simulink model "INS"  (R2018b)
settings: configuration reference "ins_config" (kept outside this file)
undefined symbols (not defined in the file): DiscIntNeverNeededParam, INS_CONST, INS_EXPORT, INS_PARAM
libraries: simulink x99, AP_Math x15, Filter x6, Quaternion x2, Rotation x2
(part 2 of 4)

== system INS/Sensor_Process/Optical_Flow_Preprocessing/Valid_Detect ==
  timestamp_ms : Inport
  vf_valid : Inport  Port=2
  Compare To Constant4 : simulink/Logic and Bit Operations/Compare To Constant  relop=<  const=100  OutDataTypeStr=uint8
  Constant : Constant  OutDataTypeStr=single
  Detect Change : simulink/Logic and Bit Operations/Detect Change  vinit=0  OutDataTypeStr=boolean
  Discrete-Time Integrator : DiscreteIntegrator  IntegratorMethod=Accumulation: Forward Euler  ExternalReset=sampled level  SampleTime=-1  OutDataTypeStr=uint32  SaturateOnIntegerOverflow=on  ICPrevOutput=DiscIntNeverNeededParam  ICPrevScaledInput=DiscIntNeverNeededParam
  Logical Operator : Logic  AllPortsSameDT=off  OutDataTypeStr=boolean
  valid : Outport
  wires:
  Compare To Constant4/1 -> Logical Operator/1
  Constant/1 -> Discrete-Time Integrator/1
  Detect Change/1 -> Discrete-Time Integrator/2
  vf_valid/1 -> Logical Operator/2
  Discrete-Time Integrator/1 -> Compare To Constant4/1
  Logical Operator/1 -> valid/1
  timestamp_ms/1 -> Detect Change/1

== system INS/Sensor_Process/Sonar_Process/Valid_Check ==
  timestamp_ms : Inport
  diatance_m : Inport  Port=2
  Translation_Data : Inport  Port=3
  Add : Sum
  Bus Selector : BusSelector  OutputSignals=vel_N_mDs,vel_E_mDs
  Compare To Constant : simulink/Logic and Bit Operations/Compare To Constant  relop=<  const=5  OutDataTypeStr=boolean
  Compare To Constant4 : simulink/Logic and Bit Operations/Compare To Constant  relop=<  const=100  OutDataTypeStr=uint8
  Constant : Constant  Value=INS_EXPORT.period  OutDataTypeStr=single
  Constant1 : Constant  OutDataTypeStr=uint8
  Delay : Delay  DelayLength=1
  Detect Change : simulink/Logic and Bit Operations/Detect Change  vinit=0  OutDataTypeStr=boolean
  Discrete-Time Integrator : DiscreteIntegrator  IntegratorMethod=Accumulation: Forward Euler  ExternalReset=sampled level  SampleTime=-1  OutDataTypeStr=uint32  SaturateOnIntegerOverflow=on  ICPrevOutput=DiscIntNeverNeededParam  ICPrevScaledInput=DiscIntNeverNeededParam
  Interval Test : simulink/Logic and Bit Operations/Interval Test  IntervalClosedRight=on  uplimit=2.5  IntervalClosedLeft=off  lowlimit=0  OutDataTypeStr=boolean
  Logical Operator : Logic  Inputs=4  AllPortsSameDT=off  OutDataTypeStr=boolean
  Sqrt : Sqrt  SaturateOnIntegerOverflow=on
  Square : Math  Operator=square  SaturateOnIntegerOverflow=on
  Square1 : Math  Operator=square  SaturateOnIntegerOverflow=on
  Switch : Switch  Criteria=u2 > Threshold
  sonar_valid : Outport
  wires:
  Detect Change/1 -> Switch/2, Discrete-Time Integrator/2
  Discrete-Time Integrator/1 -> Compare To Constant4/1
  Constant/1 -> Discrete-Time Integrator/1
  timestamp_ms/1 -> Detect Change/1
  Logical Operator/1 -> sonar_valid/1
  Constant1/1 -> Switch/1
  Switch/1 -> Delay/1
  Delay/1 -> Logical Operator/2, Switch/3
  Compare To Constant4/1 -> Logical Operator/1  "sonar_valid"
  diatance_m/1 -> Interval Test/1
  Interval Test/1 -> Logical Operator/3
  Translation_Data/1 -> Bus Selector/1
  Bus Selector/1 -> Square/1  "<vel_N_mDs>"
  Bus Selector/2 -> Square1/1  "<vel_E_mDs>"
  Square/1 -> Add/1
  Square1/1 -> Add/2
  Add/1 -> Sqrt/1
  Sqrt/1 -> Compare To Constant/1
  Compare To Constant/1 -> Logical Operator/4

== system INS/Bus_Assignment/Status_Output/INS_Flag/valid_check1 ==
  quality : Inport
  Compare To Constant : simulink/Logic and Bit Operations/Compare To Constant  relop=>=  const=time_out  OutDataTypeStr=boolean
  Compare To Constant1 : simulink/Logic and Bit Operations/Compare To Constant  relop=>  const=0  OutDataTypeStr=boolean
  Compare To Constant2 : simulink/Logic and Bit Operations/Compare To Constant  relop=>  const=0  OutDataTypeStr=boolean
  Constant : Constant  Value=INS_EXPORT.period  OutDataTypeStr=Inherit: Inherit via back propagation
  Delay : Delay  DelayLength=1
  Detect Rise Positive : simulink/Logic and Bit Operations/Detect Rise Positive  vinit=0  OutDataTypeStr=boolean
  Discrete-Time Integrator : DiscreteIntegrator  IntegratorMethod=Accumulation: Forward Euler  gainval=1  ExternalReset=level  SampleTime=-1  ICPrevOutput=DiscIntNeverNeededParam  ICPrevScaledInput=DiscIntNeverNeededParam
  Logical Operator : Logic  Operator=NOT  AllPortsSameDT=off  OutDataTypeStr=boolean
  Logical Operator1 : Logic  Operator=OR  AllPortsSameDT=off  OutDataTypeStr=boolean
  Multiply : Product
  valid : Outport
  wires:
  Multiply/1 -> valid/1
  Delay/1 -> Multiply/2, Logical Operator1/2
  Logical Operator1/1 -> Delay/1
  Detect Rise Positive/1 -> Logical Operator1/1
  Compare To Constant2/1 -> Detect Rise Positive/1
  quality/1 -> Compare To Constant1/1, Compare To Constant2/1
  Compare To Constant1/1 -> Discrete-Time Integrator/2
  Constant/1 -> Discrete-Time Integrator/1
  Discrete-Time Integrator/1 -> Compare To Constant/1
  Compare To Constant/1 -> Logical Operator/1
  Logical Operator/1 -> Multiply/1

== system INS/Bus_Assignment/Status_Output/INS_Flag/valid_check2 ==
  quality : Inport
  Compare To Constant : simulink/Logic and Bit Operations/Compare To Constant  relop=>=  const=time_out  OutDataTypeStr=boolean
  Compare To Constant1 : simulink/Logic and Bit Operations/Compare To Constant  relop=>  const=0  OutDataTypeStr=boolean
  Compare To Constant2 : simulink/Logic and Bit Operations/Compare To Constant  relop=>  const=0  OutDataTypeStr=boolean
  Constant : Constant  Value=INS_EXPORT.period  OutDataTypeStr=Inherit: Inherit via back propagation
  Delay : Delay  DelayLength=1
  Detect Rise Positive : simulink/Logic and Bit Operations/Detect Rise Positive  vinit=0  OutDataTypeStr=boolean
  Discrete-Time Integrator : DiscreteIntegrator  IntegratorMethod=Accumulation: Forward Euler  gainval=1  ExternalReset=level  SampleTime=-1  ICPrevOutput=DiscIntNeverNeededParam  ICPrevScaledInput=DiscIntNeverNeededParam
  Logical Operator : Logic  Operator=NOT  AllPortsSameDT=off  OutDataTypeStr=boolean
  Logical Operator1 : Logic  Operator=OR  AllPortsSameDT=off  OutDataTypeStr=boolean
  Multiply : Product
  valid : Outport
  wires:
  Multiply/1 -> valid/1
  Delay/1 -> Multiply/2, Logical Operator1/2
  Logical Operator1/1 -> Delay/1
  Detect Rise Positive/1 -> Logical Operator1/1
  Compare To Constant2/1 -> Detect Rise Positive/1
  quality/1 -> Compare To Constant1/1, Compare To Constant2/1
  Compare To Constant1/1 -> Discrete-Time Integrator/2
  Constant/1 -> Discrete-Time Integrator/1
  Discrete-Time Integrator/1 -> Compare To Constant/1
  Compare To Constant/1 -> Logical Operator/1
  Logical Operator/1 -> Multiply/1

== system INS/Bus_Assignment/Status_Output/INS_Flag/valid_check3 ==
  quality : Inport
  Compare To Constant : simulink/Logic and Bit Operations/Compare To Constant  relop=>=  const=time_out  OutDataTypeStr=boolean
  Compare To Constant1 : simulink/Logic and Bit Operations/Compare To Constant  relop=>  const=0  OutDataTypeStr=boolean
  Compare To Constant2 : simulink/Logic and Bit Operations/Compare To Constant  relop=>  const=0  OutDataTypeStr=boolean
  Constant : Constant  Value=INS_EXPORT.period  OutDataTypeStr=Inherit: Inherit via back propagation
  Delay : Delay  DelayLength=1
  Detect Rise Positive : simulink/Logic and Bit Operations/Detect Rise Positive  vinit=0  OutDataTypeStr=boolean
  Discrete-Time Integrator : DiscreteIntegrator  IntegratorMethod=Accumulation: Forward Euler  gainval=1  ExternalReset=level  SampleTime=-1  ICPrevOutput=DiscIntNeverNeededParam  ICPrevScaledInput=DiscIntNeverNeededParam
  Logical Operator : Logic  Operator=NOT  AllPortsSameDT=off  OutDataTypeStr=boolean
  Logical Operator1 : Logic  Operator=OR  AllPortsSameDT=off  OutDataTypeStr=boolean
  Multiply : Product
  valid : Outport
  wires:
  Multiply/1 -> valid/1
  Delay/1 -> Multiply/2, Logical Operator1/2
  Logical Operator1/1 -> Delay/1
  Detect Rise Positive/1 -> Logical Operator1/1
  Compare To Constant2/1 -> Detect Rise Positive/1
  quality/1 -> Compare To Constant1/1, Compare To Constant2/1
  Compare To Constant1/1 -> Discrete-Time Integrator/2
  Constant/1 -> Discrete-Time Integrator/1
  Discrete-Time Integrator/1 -> Compare To Constant/1
  Compare To Constant/1 -> Logical Operator/1
  Logical Operator/1 -> Multiply/1

== system INS/Bus_Assignment/Status_Output/INS_Flag/valid_check4 ==
  quality : Inport
  Compare To Constant : simulink/Logic and Bit Operations/Compare To Constant  relop=>=  const=time_out  OutDataTypeStr=boolean
  Compare To Constant1 : simulink/Logic and Bit Operations/Compare To Constant  relop=>  const=0  OutDataTypeStr=boolean
  Compare To Constant2 : simulink/Logic and Bit Operations/Compare To Constant  relop=>  const=0  OutDataTypeStr=boolean
  Constant : Constant  Value=INS_EXPORT.period  OutDataTypeStr=Inherit: Inherit via back propagation
  Delay : Delay  DelayLength=1
  Detect Rise Positive : simulink/Logic and Bit Operations/Detect Rise Positive  vinit=0  OutDataTypeStr=boolean
  Discrete-Time Integrator : DiscreteIntegrator  IntegratorMethod=Accumulation: Forward Euler  gainval=1  ExternalReset=level  SampleTime=-1  ICPrevOutput=DiscIntNeverNeededParam  ICPrevScaledInput=DiscIntNeverNeededParam
  Logical Operator : Logic  Operator=NOT  AllPortsSameDT=off  OutDataTypeStr=boolean
  Logical Operator1 : Logic  Operator=OR  AllPortsSameDT=off  OutDataTypeStr=boolean
  Multiply : Product
  valid : Outport
  wires:
  Multiply/1 -> valid/1
  Delay/1 -> Multiply/2, Logical Operator1/2
  Logical Operator1/1 -> Delay/1
  Detect Rise Positive/1 -> Logical Operator1/1
  Compare To Constant2/1 -> Detect Rise Positive/1
  quality/1 -> Compare To Constant1/1, Compare To Constant2/1
  Compare To Constant1/1 -> Discrete-Time Integrator/2
  Constant/1 -> Discrete-Time Integrator/1
  Discrete-Time Integrator/1 -> Compare To Constant/1
  Compare To Constant/1 -> Logical Operator/1
  Logical Operator/1 -> Multiply/1

== system INS/Bus_Assignment/Status_Output/INS_Flag/valid_check5 ==
  quality : Inport
  Compare To Constant : simulink/Logic and Bit Operations/Compare To Constant  relop=>=  const=time_out  OutDataTypeStr=boolean
  Compare To Constant1 : simulink/Logic and Bit Operations/Compare To Constant  relop=>  const=0  OutDataTypeStr=boolean
  Compare To Constant2 : simulink/Logic and Bit Operations/Compare To Constant  relop=>  const=0  OutDataTypeStr=boolean
  Constant : Constant  Value=INS_EXPORT.period  OutDataTypeStr=Inherit: Inherit via back propagation
  Delay : Delay  DelayLength=1
  Detect Rise Positive : simulink/Logic and Bit Operations/Detect Rise Positive  vinit=0  OutDataTypeStr=boolean
  Discrete-Time Integrator : DiscreteIntegrator  IntegratorMethod=Accumulation: Forward Euler  gainval=1  ExternalReset=level  SampleTime=-1  ICPrevOutput=DiscIntNeverNeededParam  ICPrevScaledInput=DiscIntNeverNeededParam
  Logical Operator : Logic  Operator=NOT  AllPortsSameDT=off  OutDataTypeStr=boolean
  Logical Operator1 : Logic  Operator=OR  AllPortsSameDT=off  OutDataTypeStr=boolean
  Multiply : Product
  valid : Outport
  wires:
  Multiply/1 -> valid/1
  Delay/1 -> Multiply/2, Logical Operator1/2
  Logical Operator1/1 -> Delay/1
  Detect Rise Positive/1 -> Logical Operator1/1
  Compare To Constant2/1 -> Detect Rise Positive/1
  quality/1 -> Compare To Constant1/1, Compare To Constant2/1
  Compare To Constant1/1 -> Discrete-Time Integrator/2
  Constant/1 -> Discrete-Time Integrator/1
  Discrete-Time Integrator/1 -> Compare To Constant/1
  Compare To Constant/1 -> Logical Operator/1
  Logical Operator/1 -> Multiply/1

== system INS/Bus_Assignment/Status_Output/INS_Flag/valid_check6 ==
  quality : Inport
  Compare To Constant : simulink/Logic and Bit Operations/Compare To Constant  relop=>=  const=time_out  OutDataTypeStr=boolean
  Compare To Constant1 : simulink/Logic and Bit Operations/Compare To Constant  relop=>  const=0  OutDataTypeStr=boolean
  Compare To Constant2 : simulink/Logic and Bit Operations/Compare To Constant  relop=>  const=0  OutDataTypeStr=boolean
  Constant : Constant  Value=INS_EXPORT.period  OutDataTypeStr=Inherit: Inherit via back propagation
  Delay : Delay  DelayLength=1
  Detect Rise Positive : simulink/Logic and Bit Operations/Detect Rise Positive  vinit=0  OutDataTypeStr=boolean
  Discrete-Time Integrator : DiscreteIntegrator  IntegratorMethod=Accumulation: Forward Euler  gainval=1  ExternalReset=level  SampleTime=-1  ICPrevOutput=DiscIntNeverNeededParam  ICPrevScaledInput=DiscIntNeverNeededParam
  Logical Operator : Logic  Operator=NOT  AllPortsSameDT=off  OutDataTypeStr=boolean
  Logical Operator1 : Logic  Operator=OR  AllPortsSameDT=off  OutDataTypeStr=boolean
  Multiply : Product
  valid : Outport
  wires:
  Multiply/1 -> valid/1
  Delay/1 -> Multiply/2, Logical Operator1/2
  Logical Operator1/1 -> Delay/1
  Detect Rise Positive/1 -> Logical Operator1/1
  Compare To Constant2/1 -> Detect Rise Positive/1
  quality/1 -> Compare To Constant1/1, Compare To Constant2/1
  Compare To Constant1/1 -> Discrete-Time Integrator/2
  Constant/1 -> Discrete-Time Integrator/1
  Discrete-Time Integrator/1 -> Compare To Constant/1
  Compare To Constant/1 -> Logical Operator/1
  Logical Operator/1 -> Multiply/1

== system INS/Bus_Assignment/Status_Output/INS_Flag/valid_check8 ==
  quality : Inport
  Compare To Constant : simulink/Logic and Bit Operations/Compare To Constant  relop=>=  const=time_out  OutDataTypeStr=boolean
  Compare To Constant1 : simulink/Logic and Bit Operations/Compare To Constant  relop=>  const=0  OutDataTypeStr=boolean
  Compare To Constant2 : simulink/Logic and Bit Operations/Compare To Constant  relop=>  const=0  OutDataTypeStr=boolean
  Constant : Constant  Value=INS_EXPORT.period  OutDataTypeStr=Inherit: Inherit via back propagation
  Delay : Delay  DelayLength=1
  Detect Rise Positive : simulink/Logic and Bit Operations/Detect Rise Positive  vinit=0  OutDataTypeStr=boolean
  Discrete-Time Integrator : DiscreteIntegrator  IntegratorMethod=Accumulation: Forward Euler  gainval=1  ExternalReset=level  SampleTime=-1  ICPrevOutput=DiscIntNeverNeededParam  ICPrevScaledInput=DiscIntNeverNeededParam
  Logical Operator : Logic  Operator=NOT  AllPortsSameDT=off  OutDataTypeStr=boolean
  Logical Operator1 : Logic  Operator=OR  AllPortsSameDT=off  OutDataTypeStr=boolean
  Multiply : Product
  valid : Outport
  wires:
  Multiply/1 -> valid/1
  Delay/1 -> Multiply/2, Logical Operator1/2
  Logical Operator1/1 -> Delay/1
  Detect Rise Positive/1 -> Logical Operator1/1
  Compare To Constant2/1 -> Detect Rise Positive/1
  quality/1 -> Compare To Constant1/1, Compare To Constant2/1
  Compare To Constant1/1 -> Discrete-Time Integrator/2
  Constant/1 -> Discrete-Time Integrator/1
  Discrete-Time Integrator/1 -> Compare To Constant/1
  Compare To Constant/1 -> Logical Operator/1
  Logical Operator/1 -> Multiply/1

== system INS/Data_Fusion/AHRS/Attitude_Init/Attitude_Init ==
  acc_B : Inport
  mag_B : Inport  Port=2
  Enable : EnablePort
  DCM_to_quat : Quaternion/DCM_to_quat  SystemSampleTime=-1
  Gain : Gain  Gain=-1
  Vector Concatenate : Concatenate  NumInputs=3  Mode=Multidimensional array  ConcatenateDimension=2
  cross_product : AP_Math/cross_product  SystemSampleTime=-1
  cross_product1 : AP_Math/cross_product  SystemSampleTime=-1
  safe_norm : AP_Math/safe_norm  SystemSampleTime=-1
  safe_norm1 : AP_Math/safe_norm  SystemSampleTime=-1
  safe_norm2 : AP_Math/safe_norm  SystemSampleTime=-1
  quaternion_0 : Outport  InitialOutput=[1; 0; 0; 0]
  wires:
  Gain/1 -> cross_product/1, safe_norm2/1, cross_product1/2
  acc_B/1 -> Gain/1
  Vector Concatenate/1 -> DCM_to_quat/1  "M_BO"
  cross_product1/1 -> safe_norm/1
  mag_B/1 -> cross_product/2
  cross_product/1 -> cross_product1/1, safe_norm1/1
  safe_norm1/1 -> Vector Concatenate/2  "DCM_y"
  safe_norm/1 -> Vector Concatenate/1  "DCM_x"
  safe_norm2/1 -> Vector Concatenate/3  "DCM_z"
  DCM_to_quat/1 -> quaternion_0/1

== system INS/Data_Fusion/AHRS/Attitude_Init/Onground_Check ==
  IMU_Data : Inport
  Abs : Abs
  Bus Selector : BusSelector  OutputSignals=gyr_B_radPs
  HPF : Subsystem
  LPF : Filter/LPF  T=0.5
  LPF1 : Filter/LPF  T=0.05
  MinMax1 : MinMax  Function=max
  Relay2 : Relay  OnSwitchValue=10e-3  OffSwitchValue=3e-3  OnOutputValue=0  OffOutputValue=1
  Saturation2 : Saturate  UpperLimit=1  LowerLimit=0
  Selector : Selector  InputPortWidth=3  IndexOptions=Index vector (dialog)  Indices=[1 2]  OutputSizes=1
  standstill : Outport
  wires:
  LPF1/1 -> Relay2/1
  Relay2/1 -> standstill/1
  Saturation2/1 -> LPF1/1
  HPF/1(y) -> Abs/1
  Selector/1 -> HPF/1(u)
  Abs/1 -> MinMax1/1
  LPF/1 -> Saturation2/1
  MinMax1/1 -> LPF/1  "gyr_sig"
  Bus Selector/1 -> Selector/1  "<gyr_B_radPs>"
  IMU_Data/1 -> Bus Selector/1

== system INS/Data_Fusion/AHRS/Attitude_Init/Reset_Condition ==
  IMU_valid : Inport
  Mag_valid : Inport  Port=2
  global_reset : Inport  Port=3
  acc_B_mPs2 : Inport  Port=4
  mag_norm_B : Inport  Port=5
  Compare To Constant : simulink/Logic and Bit Operations/Compare To Constant  relop=>  const=0.01  OutDataTypeStr=boolean
  Interval Test : simulink/Logic and Bit Operations/Interval Test  IntervalClosedRight=on  uplimit=INS_CONST.g+0.5  IntervalClosedLeft=on  lowlimit=INS_CONST.g-0.5  OutDataTypeStr=boolean
  Logical Operator : Logic  Operator=OR  AllPortsSameDT=off  OutDataTypeStr=boolean
  Logical Operator1 : Logic  Inputs=4  AllPortsSameDT=off  OutDataTypeStr=boolean
  reset : Subsystem
  vec_modulus : AP_Math/vec_modulus  SystemSampleTime=-1
  vec_modulus1 : AP_Math/vec_modulus  SystemSampleTime=-1
  att_reset : Outport
  wires:
  IMU_valid/1 -> Logical Operator1/1
  reset/1(reset) -> Logical Operator/1  "a_reset"
  global_reset/1 -> Logical Operator/2
  Logical Operator/1 -> att_reset/1
  Mag_valid/1 -> Logical Operator1/2
  acc_B_mPs2/1 -> vec_modulus/1
  mag_norm_B/1 -> vec_modulus1/1
  vec_modulus1/1 -> Compare To Constant/1
  Compare To Constant/1 -> Logical Operator1/4
  Interval Test/1 -> Logical Operator1/3
  vec_modulus/1 -> Interval Test/1
  Logical Operator1/1 -> reset/1(valid)  "a_valid"

== system INS/Data_Fusion/AHRS/Correct/Att_Correction ==
  Sensor_Data : Inport
  Rotation_Data : Inport  Port=2
  standstill : Inport  Port=3
  Attitude_Correct : Subsystem
  Bus Selector : BusSelector  OutputSignals=Mag_Data,GPS_Data
  Bus Selector2 : BusSelector  OutputSignals=M_BO
  Heading_Correction : Subsystem
  Multiply : Product  Multiplication=Matrix(*)
  Sum : Sum  Inputs=|++
  rot_B_correction : Outport
  wires:
  standstill/1 -> Heading_Correction/2(standstill)
  Bus Selector/1 -> Heading_Correction/3(Mag_Data)  "<Mag_Data>"
  Attitude_Correct/1(att_error_O_mPs2) -> Sum/1  "att_error_O"
  Heading_Correction/1(heading_error_O) -> Sum/2  "heading_error_O"
  Bus Selector2/1 -> Multiply/1  "<M_BO>"
  Multiply/1 -> rot_B_correction/1
  Sensor_Data/1 -> Bus Selector/1, Attitude_Correct/1(Sensor_Data)
  Sum/1 -> Multiply/2
  Bus Selector/2 -> Heading_Correction/4(GPS_Data)  "<GPS_Data>"
  Rotation_Data/1 -> Bus Selector2/1, Heading_Correction/1(Rotation_Data), Attitude_Correct/2(Rotation_Data)

== system INS/Data_Fusion/AHRS/Correct/Bias_Correction ==
  rot_B_correction : Inport
  Rotation_Data : Inport  Port=2
  standstill : Inport  Port=3
  IMU_Data : Inport  Port=4
  Abs : Abs
  Bus Selector : BusSelector  OutputSignals=acc_B_mPs2
  Bus Selector1 : BusSelector  OutputSignals=gyr_B_radDs
  Compare To Constant : simulink/Logic and Bit Operations/Compare To Constant  relop=<=  const=1  OutDataTypeStr=boolean
  Constant : Constant  Value=9.806  OutDataTypeStr=single
  Data Type Conversion : DataTypeConversion  OutDataTypeStr=single
  Gain3 : Gain  Gain=0.5
  Gain4 : Gain
  MX Product1 : Product  RndMeth=Simplest
  Onground_Correction : Subsystem
  Saturation2 : Saturate  UpperLimit=0.1/180*pi  LowerLimit=-0.1/180*pi
  Subtract : Sum  Inputs=+-
  Sum2 : Sum  Inputs=|+-
  vec_modulus : AP_Math/vec_modulus  SystemSampleTime=-1
  bias_g_correction : Outport
  wires:
  Bus Selector1/1 -> Onground_Correction/1(gyr_B_radPs)  "<gyr_B_radDs>"
  Rotation_Data/1 -> Bus Selector1/1
  standstill/1 -> Onground_Correction/2(standstill)
  IMU_Data/1 -> Bus Selector/1
  Saturation2/1 -> Sum2/1  "bias_g_correction"
  Compare To Constant/1 -> Data Type Conversion/1
  Bus Selector/1 -> vec_modulus/1  "<acc_B_mPs2>"
  MX Product1/1 -> Gain3/1
  rot_B_correction/1 -> MX Product1/1
  vec_modulus/1 -> Subtract/1
  Gain3/1 -> Saturation2/1
  Onground_Correction/1(gyr_bias) -> Gain4/1
  Gain4/1 -> Sum2/2  "rot_bias_standstil"
  Constant/1 -> Subtract/2
  Subtract/1 -> Abs/1
  Abs/1 -> Compare To Constant/1
  Data Type Conversion/1 -> MX Product1/2
  Sum2/1 -> bias_g_correction/1  "bias_g_correction"

== system INS/Data_Fusion/AHRS/Integrate/Att_Init_Done ==
  att_reset : Inport
  Constant : Constant  OutDataTypeStr=uint8
  Delay : Delay  DelayLength=1
  Detect Increase : simulink/Logic and Bit Operations/Detect Increase  vinit=0.0  OutDataTypeStr=boolean
  Switch : Switch  Criteria=u2 > Threshold
  att_init_done : Outport
  wires:
  att_reset/1 -> Detect Increase/1
  Detect Increase/1 -> Switch/2
  Constant/1 -> Switch/1
  Delay/1 -> Switch/3
  Switch/1 -> att_init_done/1, Delay/1

== system INS/Data_Fusion/AHRS/Integrate/Attitude_Integration ==
  att_reset : Inport
  quat_0 : Inport  Port=2
  rot_IB_B : Inport  Port=3
  Constant : Constant  Value=0  OutDataTypeStr=single
  Discrete-Time Integrator : DiscreteIntegrator  ExternalReset=level  InitialConditionSource=external  SampleTime=-1  ICPrevOutput=DiscIntNeverNeededParam  ICPrevScaledInput=DiscIntNeverNeededParam
  Gain2 : Gain  Gain=0.5  OutMin=-450*pi/180  OutMax=450*pi/180  RndMeth=Simplest
  Mux1 : Mux  Inputs=2
  Quat Multiply1 : Subsystem  mask(Quaternion Multiplication){}
      mask help:
      | q(1) = q1(1)*q2(1) - q1(2)*q2(2) - q1(3)*q2(3) - q1(4)*q2(4)
      | q(2) = q1(1)*q2(2) + q1(2)*q2(1) + q1(3)*q2(4) - q1(4)*q2(3)
      | q(3) = q1(1)*q2(3) - q1(2)*q2(4) + q1(3)*q2(1) + q1(4)*q2(2)
      | q(4) = q1(1)*q2(4) + q1(2)*q2(3) - q1(3)*q2(2) + q1(4)*q2(1)
      |
      | Regrettably implemented in Simulink
      mask init:
      | pos = get_param(gcb, 'Position');
      | width = pos(3) - pos(1); height = pos(4) - pos(2);
      | fontsize = get_param(gcb, 'fontsize');
      | if fontsize==-1, scale=1; else scale=fontsize/10; end
      mask Display: text(width/2-scale*14, (height/2-scale), 'q1*q2')
  Quat_to_M_OB : Rotation/Quat_to_M_OB  SystemSampleTime=-1
  Transpose2 : Math  Operator=transpose  SaturateOnIntegerOverflow=on
  quat normalize : Quaternion/quat normalize  SystemSampleTime=-1
  att_quat : Outport
  M_OB : Outport  Port=2
  M_BO : Outport  Port=3
  wires:
  Transpose2/1 -> M_BO/1
  Quat_to_M_OB/1 -> M_OB/1, Transpose2/1
  Discrete-Time Integrator/1 -> quat normalize/1
  att_reset/1 -> Discrete-Time Integrator/2
  quat_0/1 -> Discrete-Time Integrator/3
  Gain2/1 -> Discrete-Time Integrator/1
  Quat Multiply1/1(q) -> Gain2/1
  rot_IB_B/1 -> Mux1/2
  Mux1/1 -> Quat Multiply1/2(q2)
  Constant/1 -> Mux1/1
  quat normalize/1 -> Quat_to_M_OB/1, Quat Multiply1/1(q1), att_quat/1

== system INS/Data_Fusion/AHRS/Integrate/Bias_Integration ==
  bias_g_correction : Inport
  rot_IB_B : Inport  Port=2
  Discrete-Time Integrator2 : DiscreteIntegrator  SampleTime=-1  LimitOutput=on  UpperSaturationLimit=50/180*pi  LowerSaturationLimit=-50/180*pi  ICPrevOutput=DiscIntNeverNeededParam  ICPrevScaledInput=DiscIntNeverNeededParam
  Sum1 : Sum  Inputs=++|
  rot_B_cal_radDs : Outport
  bias_g : Outport  Port=2
  wires:
  bias_g_correction/1 -> Discrete-Time Integrator2/1
  Sum1/1 -> rot_B_cal_radDs/1
  Discrete-Time Integrator2/1 -> Sum1/1, bias_g/1
  rot_IB_B/1 -> Sum1/2

== system INS/Data_Fusion/AHRS/Integrate/Euler_Angle ==
  att_quat : Inport
  M_BO : Inport  Port=2
  Euler_Transformations : Subsystem
  M_CO1 : Rotation/M_CO  SystemSampleTime=-1
  Selector2 : Selector  NumberOfDimensions=2  InputPortWidth=3  IndexOptions=Index vector (dialog),Index vector (dialog)  Indices=[1 2 3],[3]  OutputSizes=1,1
  phi_rad : Outport
  theta_rad : Outport  Port=2
  psi_rad : Outport  Port=3
  M_CO : Outport  Port=4
  wires:
  Euler_Transformations/1(phi_rad) -> phi_rad/1
  Euler_Transformations/2(theta_rad) -> theta_rad/1
  Euler_Transformations/3(psi_rad) -> M_CO1/1, psi_rad/1
  M_CO1/1 -> M_CO/1
  M_BO/1 -> Selector2/1
  Selector2/1 -> Euler_Transformations/1(Oz_B)
  att_quat/1 -> Euler_Transformations/2(quat_OB)

== system INS/Data_Fusion/Translation_Filter/CF/Bus_Assignment ==
  Processed_Data : Inport
  Horizontal_States : Inport  Port=2
  Verticle_States : Inport  Port=3
  sonar_bias : Inport  Port=4
  Bus Creator : BusCreator  Inputs=12
  Constant : Constant  OutDataTypeStr=Inherit: Inherit via back propagation
  Demux1 : Demux  Outputs=3
  Demux2 : Demux  Outputs=3
  Signal_Rounting : Subsystem
  Translation_Data : Outport
  wires:
  Bus Creator/1 -> Translation_Data/1
  Demux1/3 -> Bus Creator/6  "vel_D_mDs"
  Demux1/2 -> Bus Creator/5  "vel_E_mDs"
  Demux1/1 -> Bus Creator/4  "vel_N_mDs"
  Demux2/3 -> Bus Creator/3  "h_m"
  Demux2/2 -> Bus Creator/2  "lambda_rad"
  Demux2/1 -> Bus Creator/1  "mue_rad"
  Signal_Rounting/3(ba_O_mDs2) -> Bus Creator/7  "ba_O_mDs2"
  Signal_Rounting/2(vel_O_mDs) -> Demux1/1
  Signal_Rounting/1(WGS84_Pos) -> Demux2/1
  Verticle_States/1 -> Signal_Rounting/3(Verticle_States)
  Horizontal_States/1 -> Signal_Rounting/2(Horizontal_States)
  Processed_Data/1 -> Signal_Rounting/1(Processed_Data)
  Constant/1 -> Bus Creator/12  "init_done"
  Signal_Rounting/4(h_gnd_m) -> Bus Creator/8  "h_gnd_m"
  sonar_bias/1 -> Signal_Rounting/4(sonar_bias)
  Signal_Rounting/7(h_R_m) -> Bus Creator/11  "h_R_m"
  Signal_Rounting/5(x_R_m) -> Bus Creator/9  "x_R_m"
  Signal_Rounting/6(y_R_m) -> Bus Creator/10  "y_R_m"

== system INS/Data_Fusion/Translation_Filter/CF/Horizontal_Filter ==
  Processed_Data : Inport
  Rotation_Data : Inport  Port=2
  Correct : Subsystem
  Predict : Subsystem
  Reshape : Reshape  OutputDimensionality=Customize  OutputDimensions=[6,1]
  States : Outport
  wires:
  Predict/1(X_Predict) -> Correct/1(X_Predict)
  Correct/1(X_Next) -> Reshape/1
  Reshape/1 -> Predict/1(X_Prio), States/1
  Processed_Data/1 -> Correct/2(Processed_Data), Predict/3(Processed_Data)
  Rotation_Data/1 -> Predict/2(Rotation_Data)

== system INS/Data_Fusion/Translation_Filter/CF/Verticle_Filter ==
  Processed_Data : Inport
  Rotation_Data : Inport  Port=2
  Correct : Subsystem
  Predict : Subsystem
  Reshape : Reshape  OutputDimensionality=Customize  OutputDimensions=[3,1]
  States : Outport
  wires:
  Predict/1(X_Predict) -> Correct/1(X_Predict)
  Correct/1(X_Next) -> Reshape/1
  Reshape/1 -> Predict/1(X_Prio), States/1
  Processed_Data/1 -> Correct/2(Processed_Data), Predict/3(Processed_Data)
  Rotation_Data/1 -> Predict/2(Rotation_Data)

== system INS/Data_Fusion/Translation_Filter/Process/Process_Data ==
  Sensor_Status : Inport
  Sensor_Meas : Inport  Port=2
  Rotation_Data : Inport  Port=3
  Translation_Data : Inport  Port=4
  Bus Creator : BusCreator  Inputs=4
  Bus Selector : BusSelector  OutputSignals=global_reset
  Init_Condition : Subsystem
  Sensor_Enable : Subsystem
  Sensor_Valid : Subsystem
  Proecssed_Data : Outport
  wires:
  Sensor_Enable/1(Sensor_Enable) -> Bus Creator/1  "Sensor_Enable"
  Init_Condition/1(Init_Condition) -> Bus Creator/2  "Init_Condition"
  Bus Creator/1 -> Proecssed_Data/1
  Rotation_Data/1 -> Init_Condition/4(Rotation_Data)
  Sensor_Meas/1 -> Bus Creator/3, Init_Condition/3(Sensor_Meas)  "Sensor_Meas"
  Sensor_Valid/1(Validity) -> Init_Condition/1(Validity)
  Sensor_Status/1 -> Sensor_Enable/1(Sensor_Status), Sensor_Valid/1(Sensor_Status), Bus Creator/4, Bus Selector/1  "Sensor_Status"
  Bus Selector/1 -> Init_Condition/2(global_reset)  "<global_reset>"
  Translation_Data/1 -> Init_Condition/5(Translation_Data)

== system INS/Data_Fusion/Translation_Filter/Process/Sensor_Meas ==
  Sensor_Data : Inport
  Rotation_Data : Inport  Port=2
  Baro_Process : Subsystem
  Bus Creator : BusCreator  Inputs=4
  GPS_Process : Subsystem
  OpticalFlow_Process : Subsystem
  Sonar_Process : Subsystem
  Sensor_Meas : Outport
  wires:
  Bus Creator/1 -> Sensor_Meas/1
  Sensor_Data/1 -> GPS_Process/1(Sensor_Data), Sonar_Process/1(Sensor_Data), OpticalFlow_Process/1(Sensor_Data), Baro_Process/1(Sensor_Data)
  GPS_Process/1(GPS_Meas) -> Bus Creator/1  "GPS_Meas"
  Rotation_Data/1 -> Sonar_Process/2(Rotation_Data)
  Sonar_Process/1(Sonar_Meas) -> Bus Creator/2  "Sonar_Meas"
  Baro_Process/1(Baro_Meas) -> Bus Creator/3  "Baro_Meas"
  OpticalFlow_Process/1(OptFlow_Meas) -> Bus Creator/4  "OptFlow_Meas"

== system INS/Data_Fusion/Translation_Filter/Process/Sensor_Status ==
  Sensor_Data : Inport
  Baro_Status : Subsystem
  Bus Creator : BusCreator  Inputs=5
  Bus Selector : BusSelector  OutputSignals=global_reset
  GPS_Status : Subsystem
  OpticalFlow_Status : Subsystem
  Sonar_Status : Subsystem
  Sensor_Status : Outport
  wires:
  Bus Creator/1 -> Sensor_Status/1
  Sensor_Data/1 -> GPS_Status/1(Sensor_Data), OpticalFlow_Status/1(Sensor_Data), Bus Selector/1, Baro_Status/1(Sensor_Data), Sonar_Status/1(Sensor_Data)
  GPS_Status/1(GPS_Status) -> Bus Creator/1  "GPS_Status"
  Bus Selector/1 -> Bus Creator/5  "<global_reset>"
  Sonar_Status/1(Sonar_Status) -> Bus Creator/2  "Sonar_Status"
  Baro_Status/1(Baro_Status) -> Bus Creator/3  "Baro_Status"
  OpticalFlow_Status/1(OptFlow_Status) -> Bus Creator/4  "OptFlow_Status"

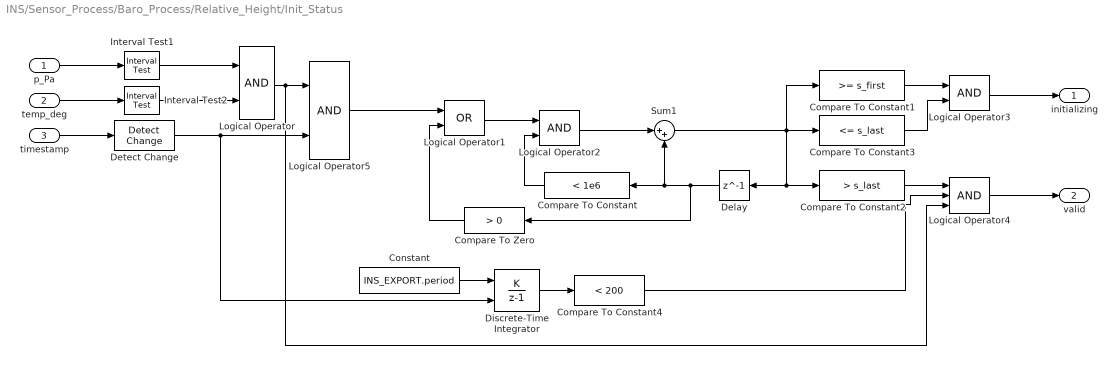
== system INS/Sensor_Process/Baro_Process/Relative_Height/Init_Status ==
  p_Pa : Inport
  temp_deg : Inport  Port=2
  timestamp : Inport  Port=3
  Compare To Constant : simulink/Logic and Bit Operations/Compare To Constant  relop=<  const=1e6  OutDataTypeStr=boolean
  Compare To Constant1 : simulink/Logic and Bit Operations/Compare To Constant  relop=>=  const=s_first  OutDataTypeStr=boolean
  Compare To Constant2 : simulink/Logic and Bit Operations/Compare To Constant  relop=>  const=s_last  OutDataTypeStr=boolean
  Compare To Constant3 : simulink/Logic and Bit Operations/Compare To Constant  relop=<=  const=s_last  OutDataTypeStr=boolean
  Compare To Constant4 : simulink/Logic and Bit Operations/Compare To Constant  relop=<  const=200  OutDataTypeStr=boolean
  Compare To Zero : simulink/Logic and Bit Operations/Compare To Zero  relop=>  OutDataTypeStr=boolean
  Constant : Constant  Value=INS_EXPORT.period  OutDataTypeStr=single
  Delay : Delay  DelayLength=1
  Detect Change : simulink/Logic and Bit Operations/Detect Change  vinit=0  OutDataTypeStr=boolean
  Discrete-Time Integrator : DiscreteIntegrator  IntegratorMethod=Accumulation: Forward Euler  ExternalReset=sampled level  SampleTime=-1  OutDataTypeStr=uint32  SaturateOnIntegerOverflow=on  ICPrevOutput=DiscIntNeverNeededParam  ICPrevScaledInput=DiscIntNeverNeededParam
  Interval Test1 : simulink/Logic and Bit Operations/Interval Test  IntervalClosedRight=off  uplimit=pressure_max  IntervalClosedLeft=off  lowlimit=pressure_min  OutDataTypeStr=boolean
  Interval Test2 : simulink/Logic and Bit Operations/Interval Test  IntervalClosedRight=off  uplimit=temp_max  IntervalClosedLeft=off  lowlimit=temp_min  OutDataTypeStr=boolean
  Logical Operator{,2..3,5} (4 alike) : Logic  AllPortsSameDT=off  OutDataTypeStr=boolean
  Logical Operator1 : Logic  Operator=OR  AllPortsSameDT=off  OutDataTypeStr=boolean
  Logical Operator4 : Logic  Inputs=3  AllPortsSameDT=off  OutDataTypeStr=boolean
  Sum1 : Sum  Inputs=|++  AccumDataTypeStr=uint32  OutDataTypeStr=uint32  RndMeth=Simplest  SaturateOnIntegerOverflow=on
  initializing : Outport
  valid : Outport  Port=2
  wires:
  Logical Operator/1 -> Logical Operator4/3, Logical Operator5/1
  Logical Operator4/1 -> valid/1
  Compare To Constant4/1 -> Logical Operator4/2
  Discrete-Time Integrator/1 -> Compare To Constant4/1
  Detect Change/1 -> Discrete-Time Integrator/2, Logical Operator5/2
  Constant/1 -> Discrete-Time Integrator/1
  Logical Operator3/1 -> initializing/1
  Compare To Constant3/1 -> Logical Operator3/2
  Compare To Constant1/1 -> Logical Operator3/1
  Compare To Constant2/1 -> Logical Operator4/1
  Compare To Constant/1 -> Logical Operator2/2
  Logical Operator1/1 -> Logical Operator2/1
  Compare To Zero/1 -> Logical Operator1/2
  Logical Operator2/1 -> Sum1/1
  Logical Operator5/1 -> Logical Operator1/1
  Sum1/1 -> Compare To Constant3/1, Compare To Constant1/1, Delay/1, Compare To Constant2/1
  Delay/1 -> Compare To Zero/1, Sum1/2, Compare To Constant/1
  Interval Test2/1 -> Logical Operator/2
  temp_deg/1 -> Interval Test2/1
  timestamp/1 -> Detect Change/1
  p_Pa/1 -> Interval Test1/1
  Interval Test1/1 -> Logical Operator/1

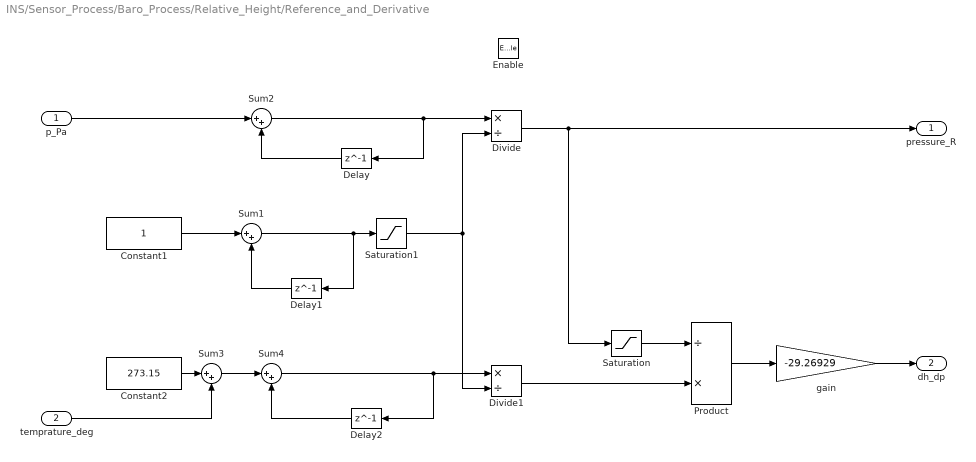
== system INS/Sensor_Process/Baro_Process/Relative_Height/Reference_and_Derivative ==
  p_Pa : Inport
  temprature_deg : Inport  Port=2
  Enable : EnablePort  StatesWhenEnabling=reset
  Constant1 : Constant  OutDataTypeStr=uint32
  Constant2 : Constant  Value=273.15  OutDataTypeStr=single
  Delay : Delay  DelayLength=1
  Delay1 : Delay  DelayLength=1
  Delay2 : Delay  DelayLength=1
  Divide : Product  Inputs=*/
  Divide1 : Product  Inputs=*/
  Product : Product  Inputs=/*
  Saturation : Saturate  UpperLimit=1200e2  LowerLimit=500
  Saturation1 : Saturate  UpperLimit=2^32  LowerLimit=1
  Sum1 : Sum  Inputs=|++  AccumDataTypeStr=uint32  OutDataTypeStr=uint32  RndMeth=Simplest  SaturateOnIntegerOverflow=on
  Sum2 : Sum  Inputs=|++
  Sum3 : Sum  Inputs=|++
  Sum4 : Sum  Inputs=|++
  gain : Gain  Gain=-29.26929
  pressure_R : Outport
  dh_dp : Outport  Port=2
  wires:
  Saturation1/1 -> Divide1/2, Divide/2
  Constant1/1 -> Sum1/1
  Sum1/1 -> Delay1/1, Saturation1/1
  Delay1/1 -> Sum1/2
  Saturation/1 -> Product/1
  Sum2/1 -> Delay/1, Divide/1
  Delay/1 -> Sum2/2
  p_Pa/1 -> Sum2/1
  Divide/1 -> pressure_R/1, Saturation/1
  Constant2/1 -> Sum3/1
  temprature_deg/1 -> Sum3/2
  Sum3/1 -> Sum4/1
  Product/1 -> gain/1
  gain/1 -> dh_dp/1
  Sum4/1 -> Delay2/1, Divide1/1
  Delay2/1 -> Sum4/2
  Divide1/1 -> Product/2

== system INS/Sensor_Process/GPS_Process/GPS_Status_and_Quality/GPS_Status ==
  note: GPS Status
      | 0: idle
      | 1: initialized, but 3D fix lost
      | 2: initialized, with 3D fix
  timeout : Inport
  hAcc : Inport  Port=2
  fixtype : Inport  Port=3
  Compare To Constant : simulink/Logic and Bit Operations/Compare To Constant  relop=<  const=5*1e3  OutDataTypeStr=uint8
  Compare To Constant1 : simulink/Logic and Bit Operations/Compare To Constant  relop===  const=3  OutDataTypeStr=uint8
  Compare To Constant2 : simulink/Logic and Bit Operations/Compare To Constant  relop=<  const=500  OutDataTypeStr=uint8
  Init_Condition : Subsystem
  Logical Operator : Logic  Inputs=3  AllPortsSameDT=off  OutDataTypeStr=fixdt(0,8)
  Logical Operator1 : Logic  Inputs=3  AllPortsSameDT=off  OutDataTypeStr=fixdt(0,8)
  Sum1 : Sum  Inputs=|++
  Status : Outport
  wires:
  Compare To Constant2/1 -> Logical Operator/3, Logical Operator1/3
  timeout/1 -> Compare To Constant2/1
  Sum1/1 -> Status/1
  Logical Operator1/1 -> Sum1/2  "3D Fix"
  hAcc/1 -> Compare To Constant/1
  Compare To Constant/1 -> Logical Operator/1
  Compare To Constant1/1 -> Logical Operator1/2, Logical Operator/2  "3D Fix"
  fixtype/1 -> Compare To Constant1/1
  Init_Condition/1(initialized) -> Sum1/1, Logical Operator1/1  "Initialize"
  Logical Operator/1 -> Init_Condition/1(valid)

== system INS/Sensor_Process/GPS_Process/GPS_Status_and_Quality/horizontal_acc ==
  hAcc : Inport
  Constant1 : Constant  Value=3  OutDataTypeStr=Inherit: Inherit via back propagation
  Gain1 : Gain  Gain=1e-3  OutDataTypeStr=single
  Gain2 : Gain  Gain=0.4  OutDataTypeStr=single
  Sum1 : Sum  Inputs=+-|
  quality : Outport
  wires:
  Sum1/1 -> Gain2/1
  Gain1/1 -> Sum1/2  "hAcc_m"
  hAcc/1 -> Gain1/1
  Constant1/1 -> Sum1/1
  Gain2/1 -> quality/1

== system INS/Sensor_Process/GPS_Process/GPS_Status_and_Quality/speed_acc ==
  sAcc : Inport
  Constant7 : Constant  Value=0.7  OutDataTypeStr=Inherit: Inherit via back propagation
  Gain3 : Gain  Gain=2.5  OutDataTypeStr=single
  Gain5 : Gain  Gain=1e-3  OutDataTypeStr=single
  Sum : Sum  Inputs=+-|
  quality : Outport
  wires:
  Gain5/1 -> Sum/2  "sAcc_m"
  Sum/1 -> Gain3/1
  sAcc/1 -> Gain5/1
  Constant7/1 -> Sum/1
  Gain3/1 -> quality/1

== system INS/Sensor_Process/GPS_Process/GPS_Status_and_Quality/timestamp_check ==
  timestamp : Inport
  Constant : Constant  Value=INS_EXPORT.period  OutDataTypeStr=single
  Detect Change : simulink/Logic and Bit Operations/Detect Change  vinit=0  OutDataTypeStr=boolean
  Discrete-Time Integrator : DiscreteIntegrator  IntegratorMethod=Accumulation: Forward Euler  ExternalReset=sampled level  SampleTime=-1  OutDataTypeStr=uint32  SaturateOnIntegerOverflow=on  UpperSaturationLimit=10000  LowerSaturationLimit=0  ICPrevOutput=DiscIntNeverNeededParam  ICPrevScaledInput=DiscIntNeverNeededParam
  timeout : Outport
  wires:
  Constant/1 -> Discrete-Time Integrator/1
  timestamp/1 -> Detect Change/1
  Detect Change/1 -> Discrete-Time Integrator/2
  Discrete-Time Integrator/1 -> timeout/1

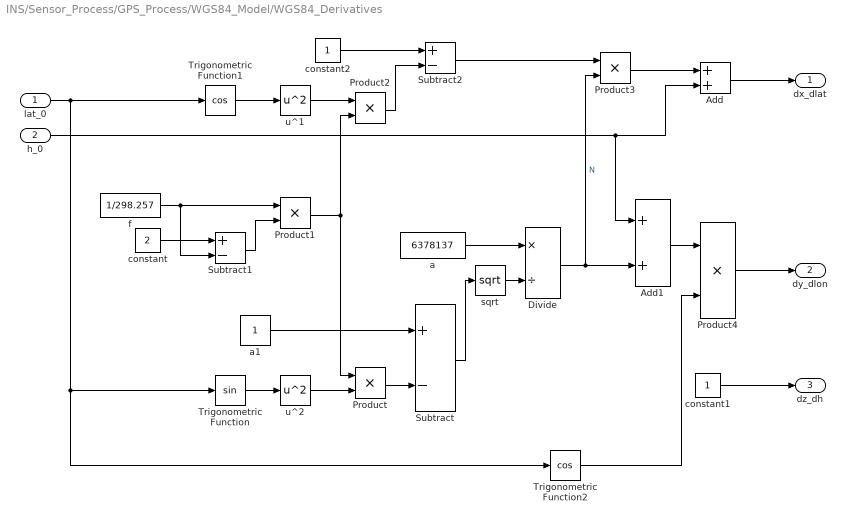
== system INS/Sensor_Process/GPS_Process/WGS84_Model/WGS84_Derivatives ==
  lat_0 : Inport
  h_0 : Inport  Port=2
  Add : Sum
  Add1 : Sum
  Divide : Product  Inputs=*/
  Product{,1..4} (5 alike) : Product  RndMeth=Zero
  Subtract : Sum  Inputs=+-
  Subtract1 : Sum  Inputs=+-
  Subtract2 : Sum  Inputs=+-
  Trigonometric Function : Trigonometry
  Trigonometric Function1 : Trigonometry  Operator=cos
  Trigonometric Function2 : Trigonometry  Operator=cos
  a : Constant  Value=6378137
  a1 : Constant
  constant : Constant  Value=2
  constant1 : Constant
  constant2 : Constant
  f : Constant  Value=1/298.257
  sqrt : Math  Operator=sqrt  SaturateOnIntegerOverflow=on
  u^1 : Math  Operator=square  SaturateOnIntegerOverflow=on
  u^2 : Math  Operator=square  SaturateOnIntegerOverflow=on
  dx_dlat : Outport
  dy_dlon : Outport  Port=2
  dz_dh : Outport  Port=3  InitialOutput=1
  wires:
  constant1/1 -> dz_dh/1
  Product4/1 -> dy_dlon/1
  Add1/1 -> Product4/1
  Trigonometric Function2/1 -> Product4/2
  Product3/1 -> Add/1
  Subtract2/1 -> Product3/1
  Product2/1 -> Subtract2/2
  u^1/1 -> Product2/1
  Trigonometric Function1/1 -> u^1/1
  constant2/1 -> Subtract2/1
  h_0/1 -> Add1/1, Add/2
  Add/1 -> dx_dlat/1
  Divide/1 -> Product3/2, Add1/2  "N"
  sqrt/1 -> Divide/2
  Product1/1 -> Product2/2, Product/1
  Subtract1/1 -> Product1/2
  constant/1 -> Subtract1/1
  f/1 -> Subtract1/2, Product1/1
  Product/1 -> Subtract/2
  Subtract/1 -> sqrt/1
  a1/1 -> Subtract/1
  u^2/1 -> Product/2
  Trigonometric Function/1 -> u^2/1
  lat_0/1 -> Trigonometric Function2/1, Trigonometric Function/1, Trigonometric Function1/1
  a/1 -> Divide/1

== system INS/Sensor_Process/IMU_Process/Bus_Assignment/IMU_Select ==
  IMU1_gyr_B_radPs : Inport
  IMU2_gyr_B_radPs : Inport  Port=2
  IMU1_acc_B_mPs2 : Inport  Port=3
  IMU2_acc_B_mPs2 : Inport  Port=4
  IMU1_Valid : Inport  Port=5
  2_Order_Butter_LPF : Filter/2_Order_Butter_LPF  wn=30*2*pi  ksi=0.707
  2_Order_Butter_LPF1 : Filter/2_Order_Butter_LPF  wn=30*2*pi  ksi=0.707
  Constant : Constant  Value=INS_PARAM.USE_EXTERN_FILTER
  Switch{,1..3} (4 alike) : Switch  Criteria=u2 > Threshold
  gyr_B_radPs : Outport
  acc_B_mPs2 : Outport  Port=2
  wires:
  IMU2_acc_B_mPs2/1 -> Switch1/3
  Switch/1 -> Switch2/1, 2_Order_Butter_LPF/1
  IMU2_gyr_B_radPs/1 -> Switch/3
  Switch1/1 -> Switch3/1, 2_Order_Butter_LPF1/1
  IMU1_gyr_B_radPs/1 -> Switch/1
  2_Order_Butter_LPF/1 -> Switch2/3
  IMU1_Valid/1 -> Switch1/2, Switch/2
  2_Order_Butter_LPF1/1 -> Switch3/3
  IMU1_acc_B_mPs2/1 -> Switch1/1
  Constant/1 -> Switch3/2, Switch2/2
  Switch2/1 -> gyr_B_radPs/1
  Switch3/1 -> acc_B_mPs2/1

== system INS/Sensor_Process/IMU_Process/Bus_Assignment/IMU_Status ==
  IMU1_valid : Inport
  IMU2_valid : Inport  Port=2
  Data Type Conversion : DataTypeConversion  OutDataTypeStr=uint8
  Gain : Gain  Gain=2  OutDataTypeStr=uint8
  Sum : Sum  Inputs=|++
  status : Outport
  wires:
  Data Type Conversion/1 -> status/1
  Gain/1 -> Sum/2
  Sum/1 -> Data Type Conversion/1
  IMU1_valid/1 -> Sum/1
  IMU2_valid/1 -> Gain/1

== system INS/Sensor_Process/IMU_Process/IMU1_Scaling/Acc_Calibrate ==
  acc_raw : Inport
  Acc_Bias : Constant  Value=INS_PARAM.AccBias  VectorParams1D=off  OutDataTypeStr=single
  Acc_RotMatrix : Constant  Value=INS_PARAM.AccRotMat  VectorParams1D=off  OutDataTypeStr=single
  Constant : Constant  Value=INS_PARAM.USE_EXTERN_FILTER
  Product5 : Product  Multiplication=Matrix(*)
  Subtract1 : Sum  Inputs=-+
  Switch : Switch  Criteria=u2 > Threshold
  acc_calib : Outport
  wires:
  Acc_RotMatrix/1 -> Product5/1
  Acc_Bias/1 -> Subtract1/1
  Product5/1 -> Switch/3
  Subtract1/1 -> Product5/2
  acc_raw/1 -> Switch/1, Subtract1/2
  Constant/1 -> Switch/2
  Switch/1 -> acc_calib/1

== system INS/Sensor_Process/IMU_Process/IMU1_Scaling/Gyro_Calibrate ==
  gyro_raw : Inport
  Constant : Constant  Value=INS_PARAM.USE_EXTERN_FILTER
  Gyr_RotMatrix : Constant  Value=INS_PARAM.GyroRotMat  VectorParams1D=off  OutDataTypeStr=single
  Gyro_Bias : Constant  Value=INS_PARAM.GyroBias  VectorParams1D=off  OutDataTypeStr=single
  Product1 : Product  Multiplication=Matrix(*)
  Subtract : Sum  Inputs=-+
  Switch : Switch  Criteria=u2 > Threshold
  gyr_calib : Outport
  wires:
  Gyro_Bias/1 -> Subtract/1
  Gyr_RotMatrix/1 -> Product1/1
  Subtract/1 -> Product1/2
  gyro_raw/1 -> Switch/1, Subtract/2
  Product1/1 -> Switch/3
  Constant/1 -> Switch/2
  Switch/1 -> gyr_calib/1

== system INS/Sensor_Process/IMU_Process/IMU2_Scaling/Acc_Calibrate ==
  acc_raw : Inport
  Acc_Bias : Constant  Value=INS_PARAM.AccBias2  VectorParams1D=off  OutDataTypeStr=single
  Acc_RotMatrix : Constant  Value=INS_PARAM.AccRotMat2  VectorParams1D=off  OutDataTypeStr=single
  Product5 : Product  Multiplication=Matrix(*)
  Subtract1 : Sum  Inputs=-+
  acc_calib : Outport
  wires:
  Acc_RotMatrix/1 -> Product5/1
  Acc_Bias/1 -> Subtract1/1
  Product5/1 -> acc_calib/1
  Subtract1/1 -> Product5/2
  acc_raw/1 -> Subtract1/2

== system INS/Sensor_Process/IMU_Process/IMU2_Scaling/Gyro_Calibrate ==
  gyro_raw : Inport
  Gyr_RotMatrix : Constant  Value=INS_PARAM.GyroRotMat2  VectorParams1D=off  OutDataTypeStr=single
  Gyro_Bias : Constant  Value=INS_PARAM.GyroBias2  VectorParams1D=off  OutDataTypeStr=single
  Product1 : Product  Multiplication=Matrix(*)
  Subtract : Sum  Inputs=-+
  gyr_calib : Outport
  wires:
  Gyro_Bias/1 -> Subtract/1
  Gyr_RotMatrix/1 -> Product1/1
  Subtract/1 -> Product1/2
  gyro_raw/1 -> Subtract/2
  Product1/1 -> gyr_calib/1

== system INS/Sensor_Process/Mag_Process/Mag_Scaling/Mag_Calibrate ==
  mag_raw : Inport
  Mag_Bias : Constant  Value=INS_PARAM.MagBias  VectorParams1D=off  OutDataTypeStr=single
  Mag_RotMatrix : Constant  Value=INS_PARAM.MagRotMat  VectorParams1D=off  OutDataTypeStr=single
  Product1 : Product  Multiplication=Matrix(*)
  Subtract : Sum  Inputs=-+
  mag_calib : Outport
  wires:
  mag_raw/1 -> Subtract/2
  Subtract/1 -> Product1/2
  Mag_RotMatrix/1 -> Product1/1
  Product1/1 -> mag_calib/1
  Mag_Bias/1 -> Subtract/1

== system INS/Sensor_Process/Mag_Process/Magnetometer/Quality_Indication ==
  note: TODO: improve this
  mag_normalized_O : Inport
  nominal_Inclination_deg : Inport  Port=2
  gps_available : Inport  Port=3
  mag_available : Inport  Port=4
  Mag_Quality_Estimate : Subsystem
  Multiply : Product  OutDataTypeStr=Inherit: Same as first input
  Switch : Switch  Criteria=u2 > Threshold
  default_mag_quality : Constant  Value=0.5  OutDataTypeStr=single
  mag_quality : Outport
  wires:
  gps_available/1 -> Switch/2
  default_mag_quality/1 -> Switch/3
  mag_available/1 -> Multiply/2
  Switch/1 -> Multiply/1
  Multiply/1 -> mag_quality/1
  nominal_Inclination_deg/1 -> Mag_Quality_Estimate/1(nominal_Inclination_deg)
  mag_normalized_O/1 -> Mag_Quality_Estimate/2(mag_normalized_O)
  Mag_Quality_Estimate/1(mag_quality) -> Switch/1

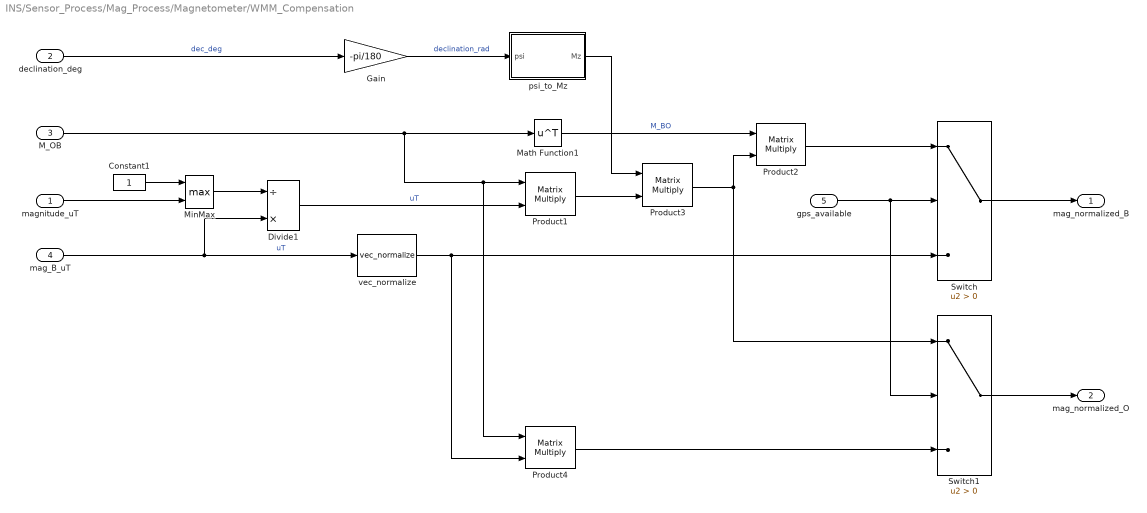
== system INS/Sensor_Process/Mag_Process/Magnetometer/WMM_Compensation ==
  magnitude_uT : Inport
  declination_deg : Inport  Port=2
  M_OB : Inport  Port=3
  mag_B_uT : Inport  Port=4
  gps_available : Inport  Port=5
  Constant1 : Constant  VectorParams1D=off  OutDataTypeStr=single
  Divide1 : Product  Inputs=/*
  Gain : Gain  Gain=-pi/180  OutDataTypeStr=single
  Math Function1 : Math  Operator=transpose  SaturateOnIntegerOverflow=on
  MinMax : MinMax  Function=max  Inputs=2
  Product{1..4} (4 alike) : Product  Multiplication=Matrix(*)
  Switch : Switch  Criteria=u2 > Threshold
  Switch1 : Switch  Criteria=u2 > Threshold
  psi_to_Mz : Subsystem
  vec_normalize : AP_Math/vec_normalize  SystemSampleTime=-1
  mag_normalized_B : Outport
  mag_normalized_O : Outport  Port=2
  wires:
  Divide1/1 -> Product1/2  "uT"
  Constant1/1 -> MinMax/1
  MinMax/1 -> Divide1/1
  magnitude_uT/1 -> MinMax/2
  psi_to_Mz/1(Mz) -> Product3/1
  Gain/1 -> psi_to_Mz/1(psi)  "declination_rad"
  declination_deg/1 -> Gain/1  "dec_deg"
  M_OB/1 -> Math Function1/1, Product1/1, Product4/1
  Math Function1/1 -> Product2/1  "M_BO"
  Product3/1 -> Product2/2, Switch1/1
  Product1/1 -> Product3/2
  mag_B_uT/1 -> Divide1/2, vec_normalize/1  "uT"
  Product2/1 -> Switch/1
  Switch/1 -> mag_normalized_B/1
  gps_available/1 -> Switch/2, Switch1/2
  vec_normalize/1 -> Switch/3, Product4/2
  Switch1/1 -> mag_normalized_O/1
  Product4/1 -> Switch1/3

== system INS/Sensor_Process/Mag_Process/Magnetometer/wmm_lookup ==
  lat_rad : Inport
  lon_rad : Inport  Port=2
  Data Type Conversion1 : DataTypeConversion  OutDataTypeStr=int32  RndMeth=Simplest
  Data Type Conversion2 : DataTypeConversion  OutDataTypeStr=int32  RndMeth=Simplest
  Declination Lookup : LookupNDDirect  Table=wmm_declination  TableDataTypeStr=int16
  Gain : Gain  Gain=180/pi/res
  Gain6 : Gain  Gain=180/pi/res
  Inclination Lookup : LookupNDDirect  Table=wmm_inclination  TableDataTypeStr=int8
  Magnitude Lookup : LookupNDDirect  Table=wmm_magnitude  TableDataTypeStr=uint8
  Saturation1 : Saturate  UpperLimit=size(wmm_magnitude,1)-1  LowerLimit=0
  Saturation2 : Saturate  UpperLimit=size(wmm_magnitude,2)-1  LowerLimit=0
  Sum : Sum  Inputs=|++
  Sum1 : Sum  Inputs=|++
  offset_lat : Constant  Value=(size(wmm_magnitude,1)-1)/2  OutDataTypeStr=int32
  offset_lon : Constant  Value=(size(wmm_magnitude,2)-1)/2  OutDataTypeStr=int32
  magnitude_uT : Outport
  declination_deg : Outport  Port=2
  inclination_deg : Outport  Port=3
  wires:
  Inclination Lookup/1 -> inclination_deg/1
  Declination Lookup/1 -> declination_deg/1
  Magnitude Lookup/1 -> magnitude_uT/1
  offset_lon/1 -> Sum1/2
  offset_lat/1 -> Sum/2
  Sum1/1 -> Saturation2/1
  Gain6/1 -> Data Type Conversion2/1
  Sum/1 -> Saturation1/1
  Gain/1 -> Data Type Conversion1/1
  Saturation2/1 -> Magnitude Lookup/2, Declination Lookup/2, Inclination Lookup/2
  Saturation1/1 -> Magnitude Lookup/1, Declination Lookup/1, Inclination Lookup/1
  lat_rad/1 -> Gain/1
  lon_rad/1 -> Gain6/1
  Data Type Conversion1/1 -> Sum/1
  Data Type Conversion2/1 -> Sum1/1

== system INS/Data_Fusion/AHRS/Attitude_Init/Onground_Check/HPF ==
  u : Inport
  LPF : Filter/LPF  T=0.25
  Sum4 : Sum  Inputs=|+-
  y : Outport
  wires:
  LPF/1 -> Sum4/2
  Sum4/1 -> y/1
  u/1 -> LPF/1, Sum4/1

== system INS/Data_Fusion/AHRS/Attitude_Init/Reset_Condition/reset ==
  valid : Inport
  Add : Sum  AccumDataTypeStr=uint32
  Data Type Conversion : DataTypeConversion  OutDataTypeStr=uint16
  Delay : Delay  DelayLength=1
  Detect Rise Positive : simulink/Logic and Bit Operations/Detect Rise Positive  vinit=0  OutDataTypeStr=boolean
  Saturation : Saturate  UpperLimit=1e3  LowerLimit=0
  valid_samples : simulink/Logic and Bit Operations/Compare To Constant  relop=>  const=50  OutDataTypeStr=boolean
  reset : Outport
  wires:
  Add/1 -> Saturation/1
  valid_samples/1 -> Detect Rise Positive/1
  Detect Rise Positive/1 -> reset/1
  Delay/1 -> Add/2
  valid/1 -> Data Type Conversion/1
  Data Type Conversion/1 -> Add/1
  Saturation/1 -> valid_samples/1, Delay/1

== system INS/Data_Fusion/AHRS/Correct/Att_Correction/Attitude_Correct ==
  Sensor_Data : Inport
  Rotation_Data : Inport  Port=2
  Acc_Correct : Subsystem
  Estimated_Acc : Subsystem
  Measured_Acc : Subsystem
  att_error_O_mPs2 : Outport
  wires:
  Measured_Acc/2(acc_ob_valid) -> Acc_Correct/2(acc_ob_valid)
  Estimated_Acc/1(acc_O_est_mPs2) -> Acc_Correct/3(acc_est_O_mPs2)  "acc_O_est_mPs2"
  Measured_Acc/3(acc_delay) -> Estimated_Acc/1(delay)
  Sensor_Data/1 -> Estimated_Acc/2(Sensor_Data), Measured_Acc/1(Sensor_Data)
  Rotation_Data/1 -> Estimated_Acc/3(Rotation_Data)
  Acc_Correct/1(att_error_O) -> att_error_O_mPs2/1
  Measured_Acc/1(meas_acc_O_mPs2) -> Acc_Correct/1(acc_meas_O_mPs2)  "acc_O_meas_mPs2"

== system INS/Data_Fusion/AHRS/Correct/Att_Correction/Heading_Correction ==
  Rotation_Data : Inport
  standstill : Inport  Port=2
  Mag_Data : Inport  Port=3
  GPS_Data : Inport  Port=4
  Bus Selector1 : BusSelector  OutputSignals=mag_norm_B,mag_quality
  Bus Selector3 : BusSelector  OutputSignals=GPS_reset
  Bus Selector4 : BusSelector  OutputSignals=M_OB
  Enable : Subsystem
  Logical Operator : Logic  Operator=OR  AllPortsSameDT=off  OutDataTypeStr=boolean
  Mag_Correction : Subsystem
  Subsystem : Subsystem
  heading_error_O : Outport
  wires:
  Bus Selector4/1 -> Subsystem/1(M_OB), Mag_Correction/1(M_OB)  "<M_OB>"
  Rotation_Data/1 -> Subsystem/3(Rotation_Data), Bus Selector4/1
  Bus Selector3/1 -> Logical Operator/2  "<GPS_reset>"
  GPS_Data/1 -> Bus Selector3/1
  Bus Selector1/2 -> Enable/1(Mag_quality)  "<mag_quality>"
  Bus Selector1/1 -> Subsystem/2(mag_B), Mag_Correction/2(mag_B)  "<mag_norm_B>"
  Mag_Data/1 -> Bus Selector1/1
  Enable/1(Mag_Correct_Enable) -> Mag_Correction/3(Mag_Correct_Enable)
  Logical Operator/1 -> Enable/2(Mag_Enable)
  standstill/1 -> Logical Operator/1
  Mag_Correction/1(mag_corr_O) -> heading_error_O/1
